simulink model "TENG_switch"  (R2016a)
settings: Solver=VariableStepAuto  StartTime=0.0  StopTime=10.0  RelTol=1e-3
libraries: fl_lib x6, elec_lib x5, nesl_utility x3, simulink x1
settings Model: Creator=mugino  LastModifiedBy=mugino

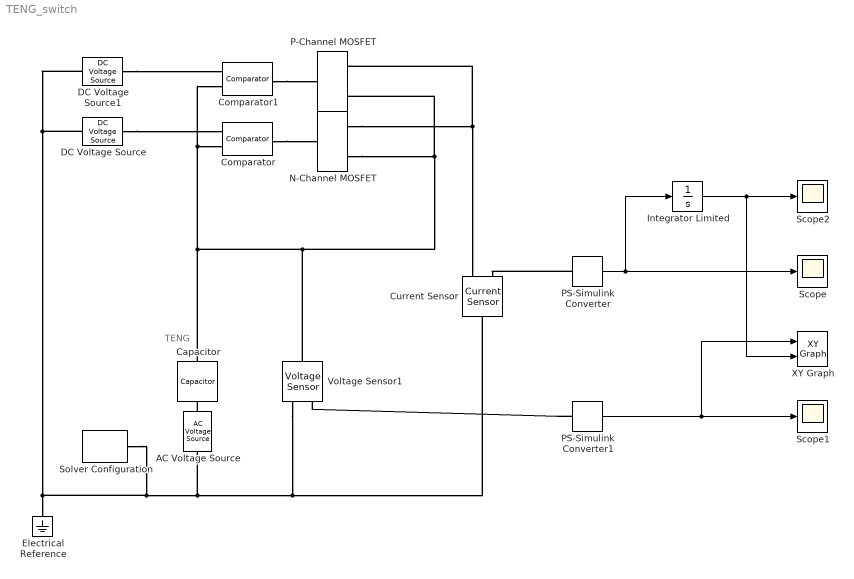
== system TENG_switch ==
  note: TENG
  AC Voltage Source : fl_lib/Electrical/Electrical Sources/AC Voltage Source  amp=110 V  shift=0 deg  frequency=1 Hz  omega=0 rad/s
  Capacitor : elec_lib/Passive Devices/Capacitor  enable_table=0  c=1e-6 F  Cvec=[ 1e-5 1e-6 ] F  Vvec=[ 0 10 ] V  CV_table_symmetry=1  C_tol=5  enable_C_tol=0  tol_distribution=1  nSigma=4  r=6 MOhm  g=0 1/Ohm  initV=0 V  enable_operating_limits=0  operating_limit_action=2  max_working_voltage_range=[ -25 25 ] V  power_rating=1 W  enable_faults=0  fault_action=1  Cscale_faulted=100  R_faulted=0.001 Ohm  G_faulted=0 1/Ohm  tau_fault=0.001 s  enable_temporal_fault=0  t_fault=1 s  enable_behavioral_fault=0  max_permissible_voltage_range=[ -100 100 ] V  t_fail_on_voltage=1 s
  Comparator : elec_lib/Integrated Circuits/Comparator  V_OS=5 V  V_OL=0 V  V_OH=5 V  C_IN=0 pF  R_OUT=60 kOhm  Delay=0 s
  Comparator1 : elec_lib/Integrated Circuits/Comparator  V_OS=5 V  V_OL=0 V  V_OH=5 V  C_IN=0 pF  R_OUT=6 Ohm  Delay=0 s
  Current Sensor : fl_lib/Electrical/Electrical Sensors/Current Sensor
  DC Voltage Source : fl_lib/Electrical/Electrical Sources/DC Voltage Source  v0=5 V
  DC Voltage Source1 : fl_lib/Electrical/Electrical Sources/DC Voltage Source  v0=-5 V
  Electrical Reference : fl_lib/Electrical/Electrical Elements/Electrical Reference
  Integrator Limited : Integrator  LimitOutput=on  UpperSaturationLimit=1  LowerSaturationLimit=0
  N-Channel MOSFET : elec_lib/Semiconductor Devices/N-Channel MOSFET  parameterization=2  prmDatasheet=1  prmEquCoeff=1  Beta=0.5 A/V^2  Rds=0.25 Ohm  Id=3e-6 A  Vgs=10 V  Vth=5 V  lam=0 1/V  Tmeas=25 degC  RS=1e-4 Ohm  RD=0.01 Ohm  C_param=1  C_GS=270 pF  C_GD=80 pF  C_DS=0 pF  C_iss=350 pF  C_rss=80 pF  C_oss=0 pF  C_GS_vec=[ 270 300 290 280 295 255 ] pF  C_GD_vec=[ 450 400 300 190 95 55 ] pF  C_DS_vec=[ 450 410 390 230 175 115 ] pF  C_iss_vec=[ 720 700 590 470 390 310 ] pF  C_rss_vec=[ 450 400 300 190 95 55 ] pF  C_oss_vec=[ 900 810 690 420 270 170 ] pF  C_Vds_vec=[ 0.1 0.3 1 3 10 30 ] V  charge_linearity_param=1  C_OX=200 pF  V_C_OX=-0.5 V  dVth_dT=-6 mV/K  Rds_T2=0.037 Ohm  Tmeas2=125 degC  BEXDatasheet=-1.5  BEXEquCoeff=-1.5  TdeviceDatasheet=25 degC  TdeviceEquCoeff=25 degC  Rth=[ 0 10 ] K/W  thermal_mass_parameterization=1  thermal_mass=[ 0 1 ] J/K  thermal_time_constant=[ 0 10 ] s  thermal_mass_initial_temperatures=[ 25 25 ] degC
  P-Channel MOSFET : elec_lib/Semiconductor Devices/P-Channel MOSFET  parameterization=2  prmDatasheet=1  prmEquCoeff=1  Beta=0.5 A/V^2  Rds=0.167 Ohm  Id=-2.5 A  Vgs=-4.5 V  Vth=-5 V  lam=0 1/V  Tmeas=25 degC  RS=1e-4 Ohm  RD=0.01 Ohm  C_param=1  C_GS=158 pF  C_GD=24 pF  C_DS=0 pF  C_iss=182 pF  C_rss=24 pF  C_oss=0 pF  C_GS_vec=[ 150 150 150 150 150 150 ] pF  C_GD_vec=[ 75 60 50 35 25 20 ] pF  C_DS_vec=[ 105 100 75 45 35 25 ] pF  C_iss_vec=[ 225 210 200 185 175 170 ] pF  C_rss_vec=[ 75 60 50 35 25 20 ] pF  C_oss_vec=[ 180 160 125 80 60 45 ] pF  C_Vsd_vec=[ 0.1 0.3 1 3 10 30 ] V  charge_linearity_param=1  C_OX=200 pF  V_C_OX=0.5 V  dVth_dT=2 mV/K  Rds_T2=0.25 Ohm  Tmeas2=125 degC  BEXDatasheet=-1.5  BEXEquCoeff=-1.5  TdeviceDatasheet=25 degC  TdeviceEquCoeff=25 degC  Rth=[ 0 10 ] K/W  thermal_mass_parameterization=1  thermal_mass=[ 0 1 ] J/K  thermal_time_constant=[ 0 10 ] s  thermal_mass_initial_temperatures=[ 25 25 ] degC
  PS-Simulink Converter : nesl_utility/PS-Simulink Converter  PhysicalDomain=network_engine_domain  SubClassName=ps_output  LeftPortType=input  RightPortType=output  PseudoPeriodic=off  Frequencies=[]  Unit=A  AffineConversion=on
  PS-Simulink Converter1 : nesl_utility/PS-Simulink Converter  PhysicalDomain=network_engine_domain  SubClassName=ps_output  LeftPortType=input  RightPortType=output  PseudoPeriodic=off  Frequencies=[]  Unit=V  AffineConversion=off
  Scope : Scope
  Scope1 : Scope
  Scope2 : Scope
  Solver Configuration : nesl_utility/Solver Configuration  PhysicalDomain=network_engine_domain  SubClassName=solver  LeftPortType=input  RightPortType=generic  Accelerate=off  Tones=[]  Harmonics=[]  SimulateNoise=off  Profile=off  UseLocalSampling=off  EnableSwitchedLinearOptims=on  FrequencyDomain=off  UseCCode=off  RelTol=0.001  AbsTol=1e-06  MinStep=1e-09  ToWorkspace=off  RevertToSquareIcSolve=off  NumHomotopyIterations=100  PhasorMode=off  PhasorModeNumHarmonics=1  OverrideAbsTol=off  DoDC=off  ResidualTolerance=1e-09  UseLocalSolver=off  LocalSolverChoice=NE_BACKWARD_EULER_ADVANCER  LocalSolverSampleTime=0.001  DoFixedCost=off  MaxNonlinIter=3  MaxModeIter=2  LinearAlgebra=Sparse  DelaysMemoryBudget=1024  AutomaticFiltering=on  FilteringTimeConstant=0.001
  Voltage Sensor1 : fl_lib/Electrical/Electrical Sensors/Voltage Sensor
  XY Graph : simulink/Sinks/XY Graph  xmin=-1  xmax=1  ymin=-1  ymax=1  st=-1
  wires:
  PS-Simulink Converter/1 -> Integrator Limited/1, Scope/1
  PS-Simulink Converter1/1 -> XY Graph/1, Scope1/1
  Integrator Limited/1 -> XY Graph/2, Scope2/1
  connections:
  AC Voltage Source/RConn1 -- Solver Configuration/RConn1 -- DC Voltage Source1/RConn1 -- DC Voltage Source/RConn1 -- Electrical Reference/LConn1 -- Current Sensor/LConn1 -- Voltage Sensor1/RConn2
  Comparator/RConn1 -- N-Channel MOSFET/LConn1
  PS-Simulink Converter1/LConn1 -- Voltage Sensor1/RConn1
  N-Channel MOSFET/RConn1 -- P-Channel MOSFET/RConn2 -- Current Sensor/RConn2
  PS-Simulink Converter/LConn1 -- Current Sensor/RConn1
  N-Channel MOSFET/RConn2 -- Voltage Sensor1/LConn1 -- Capacitor/LConn1 -- Comparator1/LConn1 -- Comparator/LConn1 -- P-Channel MOSFET/RConn1
  DC Voltage Source/LConn1 -- Comparator/LConn2
  AC Voltage Source/LConn1 -- Capacitor/RConn1
  Comparator1/RConn1 -- P-Channel MOSFET/LConn1
  DC Voltage Source1/LConn1 -- Comparator1/LConn2
